simulink model "motor_model"  (R2015b)
settings: Solver=FixedStepAuto  StartTime=0.0  StopTime=inf  FixedStep=0.0001  RelTol=1e-3
undefined symbols (not defined in the file): B, Jm, Kt, L, R
libraries: slctrlblks x1
settings Model: Creator=root  LastModifiedBy=root

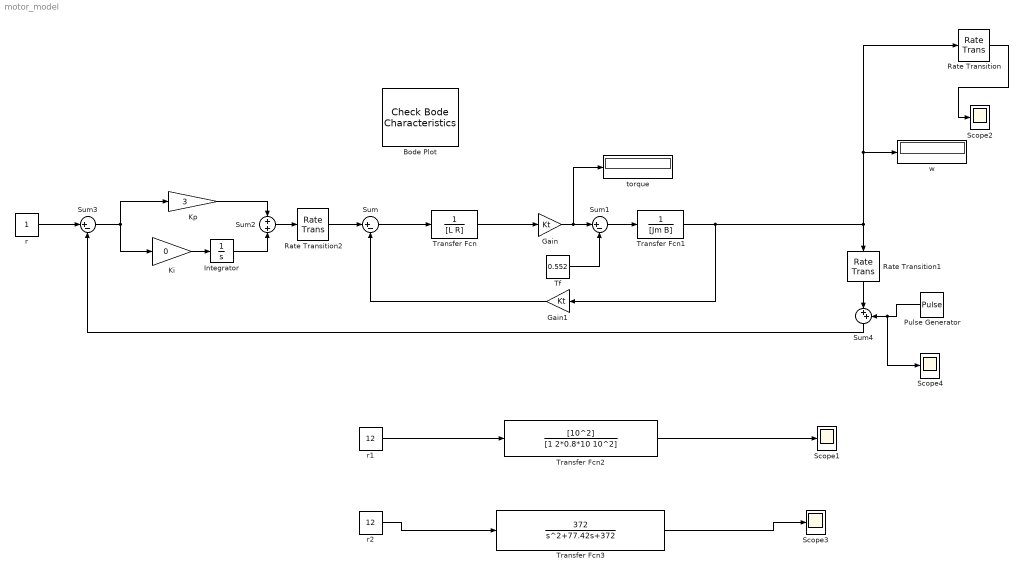
== system motor_model ==
  Bode Plot : slctrlblks/Model Verification/Check Bode  Characteristics  InstantiateOnLoad=on  SaveOperatingPoints=off  LinearizationIOs={'/Sum3', 1, 'in', 'on', '';'/Transfer Fcn1', 1, 'out', 'on', ''}  LinearizeAt=SnapshotTimes  SnapshotTimes=[0]  TriggerType=rising  SampleTime=0.0001  RateConversionMethod=zoh  PreWarpFreq=10  UseExactDelayModel=off  UseFullBlockNameLabels=off  UseBusSignalLabels=off  enabled=on  stopWhenAssertionFail=off  export=off  ViewDlgPos=[352 55 976 673]  OpenViewOnLoad=on  LaunchViewOnOpen=on  FrequencyUnits=rad/s  MagnitudeUnits=dB  PhaseUnits=deg  TimeUnits=seconds  EnableUpperBound=off  UpperBoundFrequencies=[]  UpperBoundMagnitudes=[]  EnableLowerBound=off  LowerBoundFrequencies=[]  LowerBoundMagnitudes=[]
      settings: SaveToWorkspace=on  SaveName=sys2
  Gain : Gain  Gain=Kt
  Gain1 : Gain  Gain=Kt
  Integrator : Integrator
  Ki : Gain  Gain=0
  Kp : Gain  Gain=3
  Pulse Generator : DiscretePulseGenerator  PulseType=Time based  Amplitude=0.1  Period=0.001  PulseWidth=50
  Rate Transition : RateTransition  Deterministic=off  OutPortSampleTimeOpt=Inherit  OutPortSampleTime=0.01
  Rate Transition1 : RateTransition  Deterministic=off  OutPortSampleTime=0.001
  Rate Transition2 : RateTransition  Deterministic=off  OutPortSampleTime=0.0001
  Scope{1..4} (4 alike) : Scope
  Sum : Sum  Inputs=|+-
  Sum1 : Sum  Inputs=|+-
  Sum2 : Sum  Inputs=+|+
  Sum3 : Sum  Inputs=|+-
  Sum4 : Sum  Inputs=|++
  Tf : Constant  Value=0.552
  Transfer Fcn : TransferFcn  Denominator=[L R]
  Transfer Fcn1 : TransferFcn  Denominator=[Jm B]
  Transfer Fcn2 : TransferFcn  Numerator=[10^2]  Denominator=[1 2*0.8*10 10^2]
  Transfer Fcn3 : TransferFcn  Numerator=[372]  Denominator=[1 77.42 372]
  r : Constant
  r1 : Constant  Value=12
  r2 : Constant  Value=12
  torque : Display
  w : Display
  wires:
  Sum/1 -> Transfer Fcn/1
  Gain1/1 -> Sum/2
  Transfer Fcn/1 -> Gain/1
  Tf/1 -> Sum1/2
  Sum1/1 -> Transfer Fcn1/1
  Gain/1 -> torque/1, Sum1/1
  Ki/1 -> Integrator/1
  Kp/1 -> Sum2/1
  Integrator/1 -> Sum2/2
  Sum3/1 -> Ki/1, Kp/1
  r/1 -> Sum3/1
  Sum2/1 -> Rate Transition2/1
  Rate Transition/1 -> Scope2/1
  Transfer Fcn1/1 -> Rate Transition/1, w/1, Rate Transition1/1, Gain1/1
  r1/1 -> Transfer Fcn2/1
  Transfer Fcn2/1 -> Scope1/1
  r2/1 -> Transfer Fcn3/1
  Transfer Fcn3/1 -> Scope3/1
  Sum4/1 -> Sum3/2
  Pulse Generator/1 -> Scope4/1, Sum4/2
  Rate Transition1/1 -> Sum4/1
  Rate Transition2/1 -> Sum/1
